simulink model "NH_Metrics"  (R2025b)
settings: Solver=FixedStepDiscrete  StartTime=0.0  StopTime=inf  FixedStep=0.02  RelTol=1e-3
settings Model: Creator=lolve  LastModifiedBy=lolve
settings SolverCC: AlgebraicLoopSolver=TrustRegion  DecoupledContinuousIntegration=on  MinimalZcImpactIntegration=on
settings OptimizationCC: UseDivisionForNetSlopeComputation=on
settings DebuggingCC: UnconnectedInputMsg=warning  UnconnectedOutputMsg=warning  UnconnectedLineMsg=warning  ArithmeticOperatorsInVariantConditions=warning
settings HardwareCC: ProdBitPerLong=64.0  ProdHWDeviceType=Intel->x86-64 (Linux 64)
settings ModelReferenceCC: EnableRefExpFcnMdlSchedulingChecks=on
settings SFSimCC: SimUseLocalCustomCode=off  CustomCodeUndefinedFunction=UseInterfaceOnly
settings RTWCC: SystemTargetFile=sldrt.tlc  TemplateMakefile=sldrt.tmf  RTWUseLocalCustomCode=off  RTWCompilerOptimization=on  GPUComputeCapability=3.5  DLArmComputeVersion=19.05  Description=Simulink Desktop Real-Time
settings CodeAppCC: MaxIdLength=95.0
settings SimulinkDesktopRealTimeCC: ExtModeTransport=0.0  ExtModeStaticAllocSize=1000000.0  TargetLibSuffix=_sldrt.a  TargetPreCompLibLocation=D:\MATLAB\R2025b\toolbox\sldrt\lib\win64  MultiwordLength=2048.0  DynamicStringBufferSize=256.0  ParMdlRefBuildCompliant=on  PreserveMATLABNamespacesInGeneratedCode=on  SubcomponentCodeInterfacePackaging=Reusable function  SupportVariableSizeSignals=off

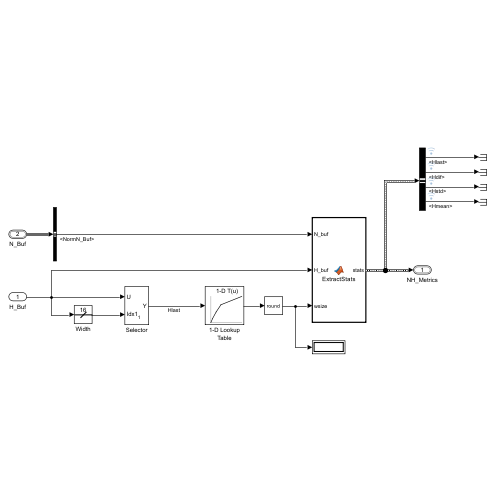
[thumbnail: Simulink's stored preview of the top-level diagram]
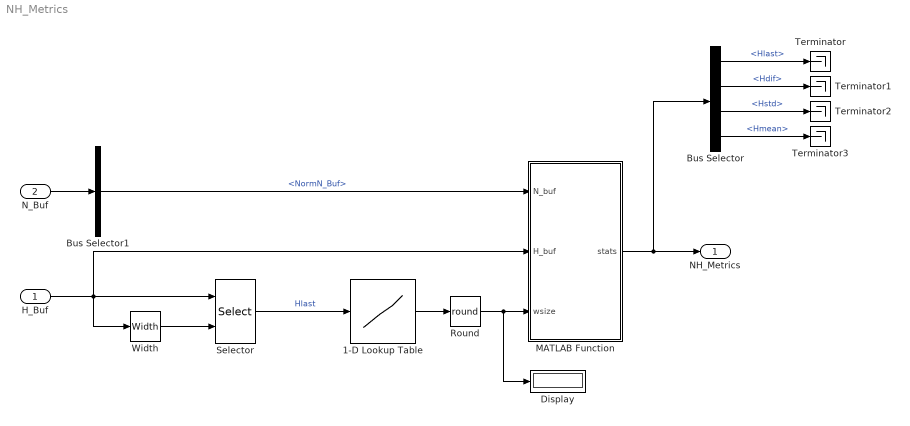
== system NH_Metrics ==
  H_Buf : Inport  OutDataTypeStr=double  PortDimensions=[16 1]
  N_Buf : Inport  Port=2  OutDataTypeStr=Bus: N_Bus_Type  PortDimensions=1
  1-D Lookup Table : Lookup_n-D  NumberOfTableDimensions=1  BreakpointsForDimension1=[0 200 500 1000 3000]  Table=[4 6 9 12 16]  ExtrapMethod=Clip  UseLastTableValue=on  InternalRulePriority=Speed  RndMeth=Simplest
  Bus Selector : BusSelector  OutputSignals=Hlast,Hdif,Hstd,Hmean
  Bus Selector1 : BusSelector  OutputSignals=NormN_Buf
  Display : Display
  MATLAB Function : MATLAB Function  TreatAsAtomicUnit=on
  Round : Rounding  Operator=round
  Selector : Selector  InputPortWidth=16  IndexOptions=Starting index (port)  Indices=[1 3]  OutputSizes=1
  Terminator{,1..3} (4 alike) : Terminator
  Width : Width  OutDataTypeMode=All ports same datatype
  NH_Metrics : Outport  OutDataTypeStr=Bus: NH_MetricsBus_Type
  wires:
  Selector/1 -> 1-D Lookup Table/1  "Hlast"
  H_Buf/1 -> MATLAB Function/2(H_buf), Width/1, Selector/1
  Bus Selector1/1 -> MATLAB Function/1(N_buf)  "<NormN_Buf>"
  Round/1 -> Display/1, MATLAB Function/3(wsize)
  Width/1 -> Selector/2
  1-D Lookup Table/1 -> Round/1
  N_Buf/1 -> Bus Selector1/1
  MATLAB Function/1(stats) -> Bus Selector/1, NH_Metrics/1
  Bus Selector/1 -> Terminator/1  "<Hlast>"
  Bus Selector/2 -> Terminator1/1  "<Hdif>"
  Bus Selector/3 -> Terminator2/1  "<Hstd>"
  Bus Selector/4 -> Terminator3/1  "<Hmean>"

== matlab function NH_Metrics/MATLAB Function ==
  data: N_buf input; H_buf input; stats output Bus: NH_MetricsBus_Type; wsize input
function stats = ExtractStats(N_buf, H_buf, wsize)
% #codegen
% =========================================================================
% НАЗНАЧЕНИЕ: Извлечение статистических метрик и динамики сигналов 
%             из кольцевых векторов истории выборок АЦП и толщин.
% =========================================================================

stats = struct(...
    'Nlast',  double(0), ...
    'Ndif',    double(0), ...
    'Nstd',   double(0), ...
    'Nmean',  double(0), ...
    'Hlast',  double(0), ...
    'Hdif',  double(0), ...
    'Hstd',   double(0), ...
    'Hmean',  double(0)...
);

stats.Hlast = H_buf(end); % последнее (мгновенное) значение толщины
stats.Nlast = N_buf(end); % последнее (мгновенное) значение кода

LastIdx = length( H_buf); % индексы начала и конца выборки
FirstIdx = LastIdx - wsize +1; % начало определяется размером окна wsize
DifIdx = LastIdx -3;
DifLen = 4;

stats.Hdif = ( H_buf( LastIdx) - H_buf( DifIdx)) / DifLen; % "скорость" изменения кодов в выборке
stats.Ndif = ( N_buf( LastIdx) - N_buf( DifIdx)) / DifLen; % "скорость" изменения толщины в выборке

stats.Hstd = std( H_buf( FirstIdx:LastIdx)); % СКО толщины в выборке
stats.Nstd = std( N_buf( FirstIdx:LastIdx)); % СКО кодов в выборке

stats.Hmean = mean( H_buf( FirstIdx:LastIdx)); % средняя толщина в выборке
stats.Nmean = mean( N_buf( FirstIdx:LastIdx)); % средний код в выборке
